simulink model "Arduino_Simulink_CarController"  (R2018a)
settings: Solver=FixedStepAuto  StartTime=0.0  StopTime=inf  RelTol=1e-3  EnableMultiTasking=on
libraries: arduinolib x6
settings Model: SimulationMode=external  ExtModeTrigDuration=2  Creator=DELL  LastModifiedBy=DELL
settings OptimizationCC: LifeSpan=Inf  MaxStackSize=64
settings DebuggingCC: SFUnexpectedBacktrackingDiag=warning  SFNoUnconditionalDefaultTransitionDiag=warning  SFExecutionAtInitializationDiag=none
settings HardwareCC: ProdBitPerInt=16  ProdBitPerPointer=16  ProdBitPerSizeT=16  ProdBitPerPtrDiffT=16  ProdLargestAtomicFloat=None  ProdWordSize=8  ProdHWDeviceType=Atmel->AVR
settings SFSimCC: MATLABDynamicMemAlloc=off
settings RTWCC: SystemTargetFile=ert.tlc  HardwareBoard=Arduino Uno  TLCOptions=-aInlineSetEventsForThisBaseRateFcn=TLC_FALSE -aSuppressMultiTaskScheduler=TLC_FALSE -aRateBasedStepFcn=1  TemplateMakefile=ert_default_tmf  GenerateReport=on  Toolchain=Arduino AVR  BuildConfiguration=Faster Runs  IncludeHyperlinkInReport=on  LaunchReport=on  GenerateTraceInfo=on  GenerateTraceReport=on  GenerateTraceReportSl=on  GenerateTraceReportSf=on  GenerateTraceReportEml=on
settings CodeAppCC: ForceParamTrailComments=on  IgnoreCustomStorageClasses=off  OperatorAnnotations=on  SimulinkDataObjDesc=on  SFDataObjDesc=on  MATLABFcnDesc=on  InsertBlockDesc=on  StateflowObjectComments=on  MATLABSourceComments=on
settings ERTTargetCC: MultiwordLength=2048  SupportContinuousTime=on  SupportVariableSizeSignals=on
settings ConfigComp: CovMetricSettings=dw  CovHtmlReporting=on  CovSaveCumulativeToWorkspaceVar=on  CovSaveSingleToWorkspaceVar=on  CovExternalEMLEnable=off

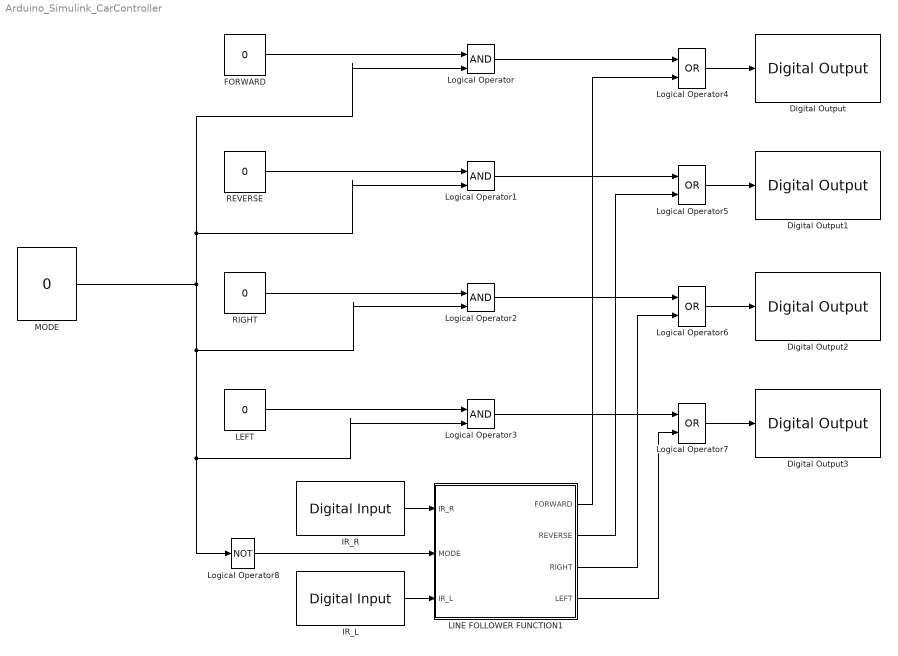
== system Arduino_Simulink_CarController ==
  Digital Output : arduinolib/Digital Output  pinNumber=12  blockPlatform=arduino
  Digital Output1 : arduinolib/Digital Output  pinNumber=13  blockPlatform=arduino
  Digital Output2 : arduinolib/Digital Output  pinNumber=8  blockPlatform=arduino
  Digital Output3 : arduinolib/Digital Output  pinNumber=9  blockPlatform=arduino
  FORWARD : Constant  Value=0
  IR_L : arduinolib/Digital Input  pinNumber=11  sampleTime=1  blockPlatform=arduino
      settings: SourceProductName=Simulink Support Package for Arduino Hardware
  IR_R : arduinolib/Digital Input  pinNumber=10  sampleTime=1  blockPlatform=arduino
      settings: SourceProductName=Simulink Support Package for Arduino Hardware
  LEFT : Constant  Value=0
  LINE FOLLOWER FUNCTION1 : MATLAB Function  TreatAsAtomicUnit=on
  Logical Operator{,1..3} (4 alike) : Logic  IconShape=distinctive  AllPortsSameDT=off  OutDataTypeStr=boolean
  Logical Operator{4..7} (4 alike) : Logic  Operator=OR  IconShape=distinctive  AllPortsSameDT=off  OutDataTypeStr=boolean
  Logical Operator8 : Logic  Operator=NOT  IconShape=distinctive  AllPortsSameDT=off  OutDataTypeStr=boolean
  MODE : Constant  Value=0
  REVERSE : Constant  Value=0
  RIGHT : Constant  Value=0
  wires:
  FORWARD/1 -> Logical Operator/1
  REVERSE/1 -> Logical Operator1/1
  RIGHT/1 -> Logical Operator2/1
  LEFT/1 -> Logical Operator3/1
  MODE/1 -> Logical Operator/2, Logical Operator1/2, Logical Operator3/2, Logical Operator8/1, Logical Operator2/2
  Logical Operator/1 -> Logical Operator4/1
  Logical Operator5/1 -> Digital Output1/1
  Logical Operator4/1 -> Digital Output/1
  Logical Operator7/1 -> Digital Output3/1
  Logical Operator6/1 -> Digital Output2/1
  Logical Operator1/1 -> Logical Operator5/1
  Logical Operator2/1 -> Logical Operator6/1
  Logical Operator3/1 -> Logical Operator7/1
  IR_R/1 -> LINE FOLLOWER FUNCTION1/1(IR_R)
  IR_L/1 -> LINE FOLLOWER FUNCTION1/3(IR_L)
  Logical Operator8/1 -> LINE FOLLOWER FUNCTION1/2(MODE)
  LINE FOLLOWER FUNCTION1/1(FORWARD) -> Logical Operator4/2
  LINE FOLLOWER FUNCTION1/2(REVERSE) -> Logical Operator5/2
  LINE FOLLOWER FUNCTION1/3(RIGHT) -> Logical Operator6/2
  LINE FOLLOWER FUNCTION1/4(LEFT) -> Logical Operator7/2

== matlab function Arduino_Simulink_CarController/LINE FOLLOWER FUNCTION1 ==
  data: FORWARD output; IR_R input; REVERSE output; MODE input; IR_L input; RIGHT output; LEFT output
function [FORWARD,REVERSE,RIGHT,LEFT] = LINE_FOLLOWER(IR_R,MODE,IR_L)
%#codegen

% at normal case the Digital O/P from sensor = 1
% any surface that reflects light will trigger sensor O/P to = 0
% the only surface that abbsorbs all radiation is a Black surface 
% the sensor will not detect black surface(esraa), so O/P will be 1 
while MODE == 1
   % Normal Case, no black surface detected
    if IR_R == 0 && IR_L == 0
    FORWARD = 1;
    REVERSE = 0;
    % black surface detected by Right IR senor
    elseif IR_R == 1 && IR_L == 0
    LEFT = 1;
    RIGHT = 0;
    FORWARD = 1;
    REVERSE = 0;
    % black surface detected by Left IR senor
    elseif IR_R == 0 && IR_L == 1
    LEFT = 0;
    RIGHT = 1;
    FORWARD = 1;
    REVERSE = 0;
    % stop
    else 
    FORWARD = 0;
    REVERSE = 0;       
    end    
end    

end
